simulink model "Final_16_12_24_simu"  (R2021a)
settings: Solver=VariableStepAuto  StartTime=0.0  StopTime=50  RelTol=1e-3
values from neighbouring files (symbols this model uses):
  K = Ka(1:3)    [Final_16_12_24.m]
  ki = - Ka(end)    [Final_16_12_24.m]
  ue = 1    [Final_16_12_24.m]
  xe = [2; 1; 1]    [Final_16_12_24.m]
  ye = 1    [Final_16_12_24.m]
libraries: cstblocks x2
settings Model: Creator=Santiago  LastModifiedBy=Santiago

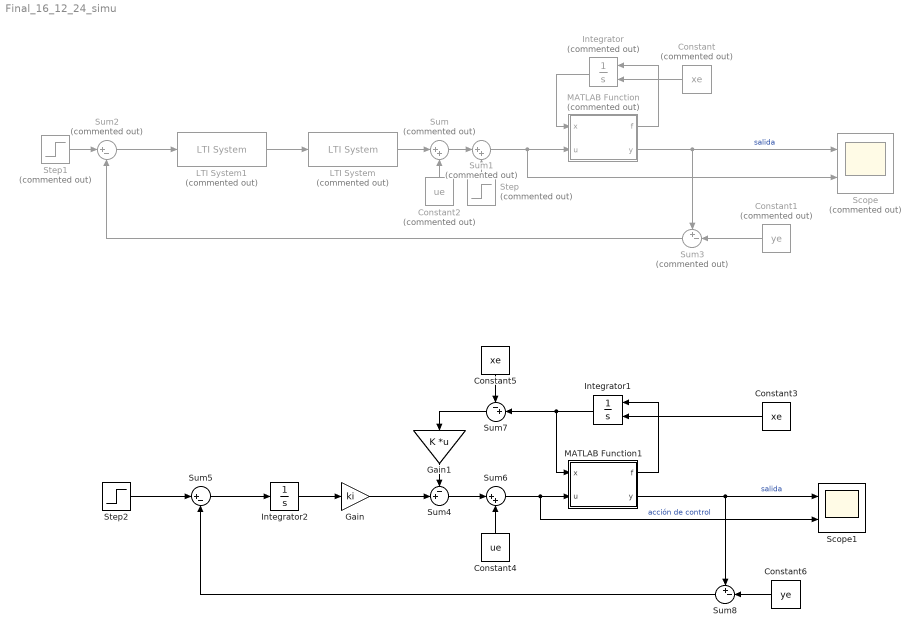
== system Final_16_12_24_simu ==
  Constant : Constant  Commented=on  Value=xe
  Constant1 : Constant  Commented=on  Value=ye
  Constant2 : Constant  Commented=on  Value=ue
  Constant3 : Constant  Value=xe
  Constant4 : Constant  Value=ue
  Constant5 : Constant  Value=xe
  Constant6 : Constant  Value=ye
  Gain : Gain  Gain=ki
  Gain1 : Gain  Gain=K  Multiplication=Matrix(K*u) (u vector)
  Integrator : Integrator  Commented=on  InitialConditionSource=external
  Integrator1 : Integrator  InitialConditionSource=external
  Integrator2 : Integrator
  LTI System : cstblocks/LTI System  Commented=on  sys=H  IC=[]
  LTI System1 : cstblocks/LTI System  Commented=on  sys=C_dig  IC=[]
  MATLAB Function : MATLAB Function  Commented=on  TreatAsAtomicUnit=on
  MATLAB Function1 : MATLAB Function  TreatAsAtomicUnit=on
  Scope : Scope  Commented=on  NumInputPorts=2
  Scope1 : Scope  NumInputPorts=2
  Step : Step  Commented=on  Time=10  After=0.1  SampleTime=0
  Step1 : Step  Commented=on  After=0.1  SampleTime=0
  Step2 : Step  After=0.1  SampleTime=0
  Sum : Sum  Commented=on  Inputs=|++
  Sum1 : Sum  Commented=on  Inputs=|++
  Sum2 : Sum  Commented=on  Inputs=|+-
  Sum3 : Sum  Commented=on  Inputs=+-|
  Sum4 : Sum  Inputs=-+|
  Sum5 : Sum  Inputs=|+-
  Sum6 : Sum  Inputs=|++
  Sum7 : Sum  Inputs=-+|
  Sum8 : Sum  Inputs=+-|
  wires:
  MATLAB Function/2(y) -> Sum3/1, Scope/1  "salida"
  Constant1/1 -> Sum3/2
  Sum3/1 -> Sum2/2
  Sum2/1 -> LTI System1/1
  MATLAB Function/1(f) -> Integrator/1
  Integrator/1 -> MATLAB Function/1(x)
  Constant/1 -> Integrator/2
  Step1/1 -> Sum2/1
  LTI System1/1 -> LTI System/1
  LTI System/1 -> Sum/1
  Constant2/1 -> Sum/2
  Sum/1 -> Sum1/1
  Sum1/1 -> Scope/2, MATLAB Function/2(u)
  Step/1 -> Sum1/2
  Integrator1/1 -> Sum7/2, MATLAB Function1/1(x)
  MATLAB Function1/1(f) -> Integrator1/1
  Constant3/1 -> Integrator1/2
  Integrator2/1 -> Gain/1
  Gain1/1 -> Sum4/1
  Gain/1 -> Sum4/2
  MATLAB Function1/2(y) -> Sum8/1, Scope1/1  "salida"
  Sum5/1 -> Integrator2/1
  Sum4/1 -> Sum6/1
  Step2/1 -> Sum5/1
  Sum7/1 -> Gain1/1
  Constant4/1 -> Sum6/2
  Constant5/1 -> Sum7/1
  Sum6/1 -> Scope1/2, MATLAB Function1/2(u)  "acción de control"
  Sum8/1 -> Sum5/2
  Constant6/1 -> Sum8/2

== matlab function Final_16_12_24_simu/MATLAB Function ==
  data: x input; f output; u input; y output
function [f, y] = fcn(x, u)
x1 = x(1);
x2 = x(2);

f1 = (-sqrt(x1 - x2) + u)/x1^2;
f2 = (sqrt(x1 - x2) - sqrt(x2))/x2^2;
f = [f1; f2];

y = x2;

== matlab function Final_16_12_24_simu/MATLAB Function1 ==
  data: x input; f output; u input; y output
function [f, y] = fcn(x, u)
x1 = x(1);
x2 = x(2);
x3 = x(3);

f1 = (-sqrt(x1 - x2) + x3)/x1^2;
f2 = (sqrt(x1 - x2) - sqrt(x2))/x2^2;
f3 = -0.02 * x3 + 0.02 * u;
f = [f1; f2; f3];

y = x2;
